simulink model "questao3_4_simu"  (R2024b)
settings: Solver=VariableStepAuto  StartTime=0.0  StopTime=100  RelTol=1e-3
values from neighbouring files (symbols this model uses):
  A = [0,   0,   1,    0 ... (first row only)    [projeto_final.m]    (also in questao3_4.m)
  B = [ 0; 0; 1/mc;  1/(L*mc)]    [projeto_final.m]    (also in questao3_4.m = [0; 0; 1/mc;  1/(L*mc)])
  N_ = Nu + K * Nx    [questao3_4.m]
undefined symbols (not defined in the file or in its folder): K
settings Model: Creator=bruno  LastModifiedBy=bruno

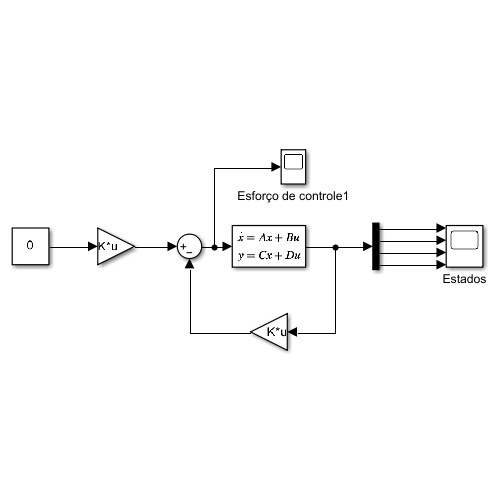
[thumbnail: Simulink's stored preview of the top-level diagram]
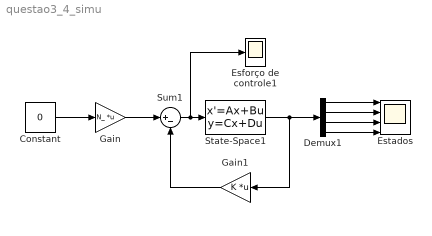
== system questao3_4_simu ==
  Constant : Constant  Value=0
  Demux1 : Demux
  Esforço de controle1 : Scope
  Estados : Scope  NumInputPorts=4
  Gain : Gain  Gain=N_  Multiplication=Matrix(K*u)
  Gain1 : Gain  Gain=K  Multiplication=Matrix(K*u)
  State-Space1 : StateSpace  A=A  B=B  C=[1,0,0,0; 0,1,0,0; 0,0,1,0; 0,0,0,1]  D=[0;0;0;0]  InitialCondition=[0, 10, 0, 0]
  Sum1 : Sum  Inputs=|+-
  wires:
  State-Space1/1 -> Demux1/1, Gain1/1
  Gain/1 -> Sum1/1
  Sum1/1 -> Esforço de controle1/1, State-Space1/1
  Gain1/1 -> Sum1/2
  Demux1/1 -> Estados/1
  Demux1/2 -> Estados/2
  Demux1/3 -> Estados/3
  Demux1/4 -> Estados/4
  Constant/1 -> Gain/1
